simulink model "Reed_solomon"  (R2013a)
settings: Solver=ode45  StartTime=0.0  StopTime=500  RelTol=1e-3
undefined symbols (not defined in the file or in its folder): rsgenpoly
libraries: commblkcod2 x2, commrandsrc2 x1
settings Model: Creator=CQ42  LastModifiedBy=OSC unnes

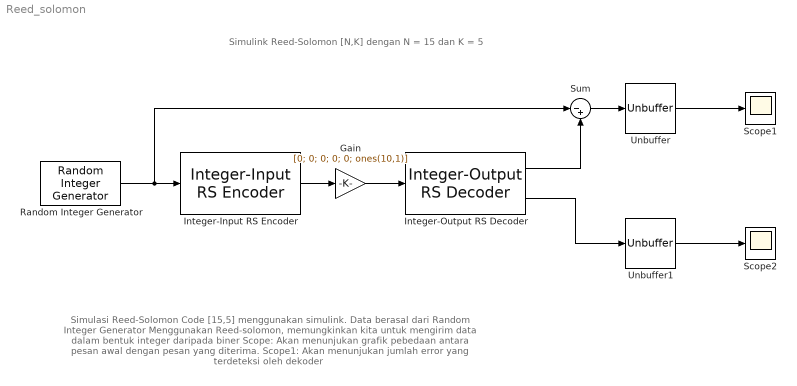
== system Reed_solomon ==
  note: Simulasi Reed-Solomon Code [15,5] menggunakan simulink. Data berasal dari Random Integer Generator
      | Menggunakan Reed-solomon, memungkinkan kita untuk mengirim data dalam bentuk integer daripada biner
      |
      | Scope: Akan menunjukan grafik pebedaan antara pesan awal dengan pesan yang diterima.
      | Scope1: Akan menunjukan jumlah error yang terdeteksi oleh dekoder
  note: Simulink Reed-Solomon [N,K] dengan N = 15 dan K = 5
  Gain : Gain  Gain=[0; 0; 0; 0; 0; ones(10,1)]
  Integer-Input RS Encoder : commblkcod2/Integer-Input RS Encoder  n=15  k=5  specPrimPoly=off  prPoly=[1 0 1 1]  specGenPoly=off  genPoly=rsgenpoly(7,3)  specPuncture=off  punctVec=[ones(2,1); zeros(2,1)]
  Integer-Output RS Decoder : commblkcod2/Integer-Output RS Decoder  n=15  k=5  specPrimPoly=off  prPoly=[1 0 1 1]  specGenPoly=off  genPoly=rsgenpoly(7,3)  specPuncture=off  punctVec=[ones(2,1); zeros(2,1)]  specErasurePort=off  showNumErr=on
  Random Integer Generator : commrandsrc2/Random Integer Generator  mul=15  seed=40813  Ts=1  frameBased=on  sampPerFrame=5  orient=off  outDataType=double
  Scope1 : Scope
  Scope2 : Scope
      settings: YMin=0  YMax=6
  Sum : Sum  Inputs=|-+
  Unbuffer : Unbuffer  SampleBasedProcessing=Same as frame based
  Unbuffer1 : Unbuffer  SampleBasedProcessing=Same as frame based
  wires:
  Integer-Input RS Encoder/1 -> Gain/1
  Gain/1 -> Integer-Output RS Decoder/1
  Integer-Output RS Decoder/1 -> Sum/2
  Sum/1 -> Unbuffer/1
  Integer-Output RS Decoder/2 -> Unbuffer1/1
  Unbuffer1/1 -> Scope2/1
  Unbuffer/1 -> Scope1/1
  Random Integer Generator/1 -> Sum/1, Integer-Input RS Encoder/1
